simulink library "CTRL_LO"  (R2023b)
settings: Solver=VariableStepAuto  StartTime=0.0  StopTime=10.0  RelTol=1e-3
undefined symbols (not defined in the file or in its folder): CTRL_LO_p_SwtTqMotReqStrat_na
libraries: CTRL_LO_FRDIST x1, CTRL_LO_ST1 x1, CTRL_LO_ST2 x1, CTRL_LO_ST3 x1, CTRL_LO_ST4 x1, CTRL_LO_ST5 x1
settings Model: Creator=blatak  LastModifiedBy=blatak

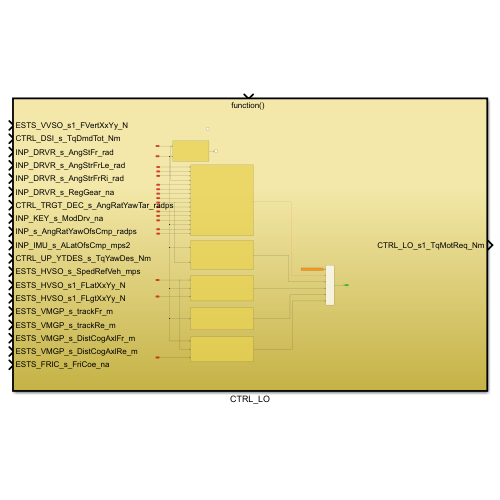
[thumbnail: Simulink's stored preview of the top-level diagram]
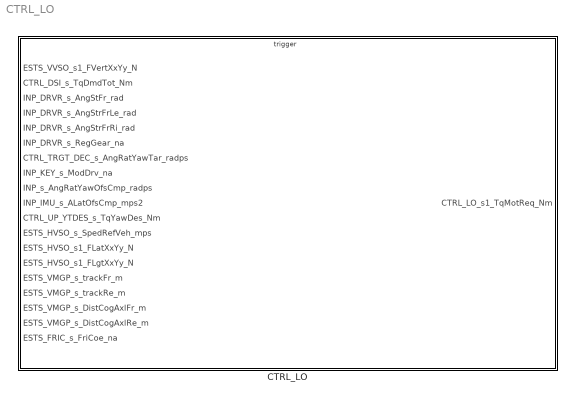
== system CTRL_LO ==
  CTRL_LO : Subsystem  TreatAsAtomicUnit=on

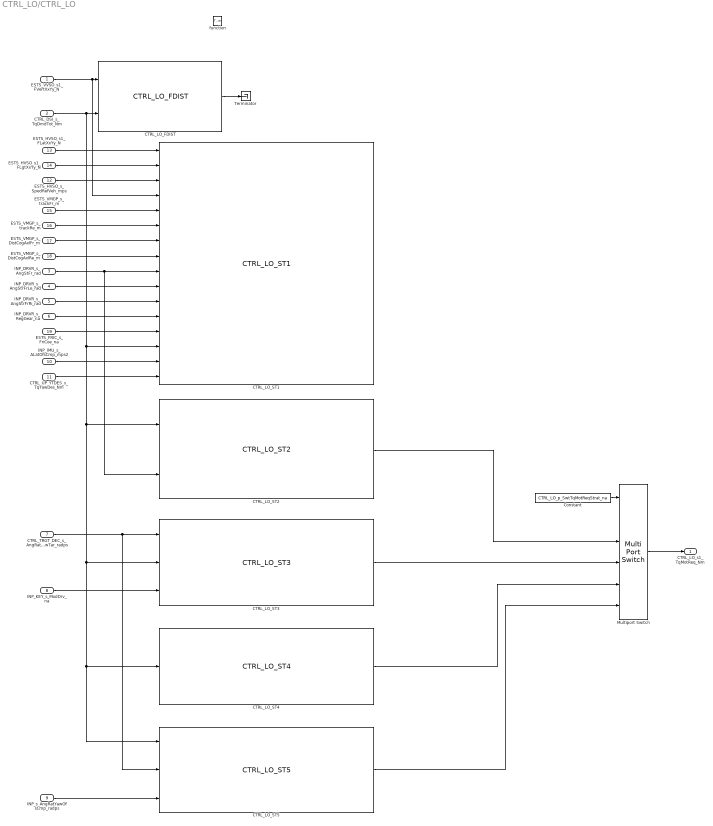
== system CTRL_LO/CTRL_LO ==
  ESTS_VVSO_s1_FVertXxYy_N : Inport
  CTRL_DSI_s_TqDmdTot_Nm : Inport  Port=2
  INP_DRVR_s_AngStFr_rad : Inport  Port=3
  INP_DRVR_s_AngStrFrLe_rad : Inport  Port=4
  INP_DRVR_s_AngStrFrRi_rad : Inport  Port=5
  INP_DRVR_s_RegGear_na : Inport  Port=6
  CTRL_TRGT_DEC_s_AngRatYawTar_radps : Inport  Port=7
  INP_KEY_s_ModDrv_na : Inport  Port=8
  INP_s_AngRatYawOfsCmp_radps : Inport  Port=9
  INP_IMU_s_ALatOfsCmp_mps2 : Inport  Port=10
  CTRL_UP_YTDES_s_TqYawDes_Nm : Inport  Port=11
  ESTS_HVSO_s_SpedRefVeh_mps : Inport  Port=12
  ESTS_HVSO_s1_FLatXxYy_N : Inport  Port=13
  ESTS_HVSO_s1_FLgtXxYy_N : Inport  Port=14
  ESTS_VMGP_s_trackFr_m : Inport  Port=15
  ESTS_VMGP_s_trackRe_m : Inport  Port=16
  ESTS_VMGP_s_DistCogAxlFr_m : Inport  Port=17
  ESTS_VMGP_s_DistCogAxlRe_m : Inport  Port=18
  ESTS_FRIC_s_FriCoe_na : Inport  Port=19
  function : TriggerPort  TriggerType=function-call  VariantControl=(inherit)
  CTRL_LO_FDIST : CTRL_LO_FRDIST/CTRL_LO_FDIST  SystemSampleTime=-1  VariantActivationTime=update diagram  AllowFlexibleInterface=on  Latency=0  AutoFrameSizeCalculation=off
  CTRL_LO_ST1 : CTRL_LO_ST1/CTRL_LO_ST1  SystemSampleTime=-1  VariantActivationTime=update diagram  AllowFlexibleInterface=on  Latency=0  AutoFrameSizeCalculation=off
  CTRL_LO_ST2 : CTRL_LO_ST2/CTRL_LO_ST2  SystemSampleTime=-1  VariantActivationTime=update diagram  AllowFlexibleInterface=on  Latency=0  AutoFrameSizeCalculation=off
  CTRL_LO_ST3 : CTRL_LO_ST3/CTRL_LO_ST3  SystemSampleTime=-1  VariantActivationTime=update diagram  AllowFlexibleInterface=on  Latency=0  AutoFrameSizeCalculation=off
  CTRL_LO_ST4 : CTRL_LO_ST4/CTRL_LO_ST4  SystemSampleTime=-1  VariantActivationTime=update diagram  AllowFlexibleInterface=on  Latency=0  AutoFrameSizeCalculation=off
  CTRL_LO_ST5 : CTRL_LO_ST5/CTRL_LO_ST5  SystemSampleTime=-1  VariantActivationTime=update diagram  AllowFlexibleInterface=on  Latency=0  AutoFrameSizeCalculation=off
  Constant : Constant  Value=CTRL_LO_p_SwtTqMotReqStrat_na
  Multiport Switch : MultiPortSwitch  Inputs=5  SaturateOnIntegerOverflow=off  InputSameDT=off
  Terminator : Terminator
  CTRL_LO_s1_TqMotReq_Nm : Outport
  wires:
  ESTS_VVSO_s1_FVertXxYy_N/1 -> CTRL_LO_ST1/4, CTRL_LO_FDIST/1
  CTRL_DSI_s_TqDmdTot_Nm/1 -> CTRL_LO_ST5/1, CTRL_LO_ST4/1, CTRL_LO_ST3/2, CTRL_LO_ST2/1, CTRL_LO_ST1/14, CTRL_LO_FDIST/2
  CTRL_LO_FDIST/1 -> Terminator/1
  ? -> Multiport Switch/2
  CTRL_LO_ST2/1 -> Multiport Switch/3
  CTRL_LO_ST3/1 -> Multiport Switch/4
  CTRL_LO_ST4/1 -> Multiport Switch/5
  CTRL_LO_ST5/1 -> Multiport Switch/6
  Multiport Switch/1 -> CTRL_LO_s1_TqMotReq_Nm/1
  INP_DRVR_s_AngStFr_rad/1 -> CTRL_LO_ST2/2, CTRL_LO_ST1/9
  CTRL_TRGT_DEC_s_AngRatYawTar_radps/1 -> CTRL_LO_ST5/2, CTRL_LO_ST3/1
  INP_KEY_s_ModDrv_na/1 -> CTRL_LO_ST3/3
  INP_s_AngRatYawOfsCmp_radps/1 -> CTRL_LO_ST5/3
  Constant/1 -> Multiport Switch/1
  CTRL_UP_YTDES_s_TqYawDes_Nm/1 -> CTRL_LO_ST1/16
  ESTS_HVSO_s1_FLatXxYy_N/1 -> CTRL_LO_ST1/1
  ESTS_HVSO_s1_FLgtXxYy_N/1 -> CTRL_LO_ST1/2
  ESTS_HVSO_s_SpedRefVeh_mps/1 -> CTRL_LO_ST1/3
  ESTS_VMGP_s_trackFr_m/1 -> CTRL_LO_ST1/5
  ESTS_VMGP_s_trackRe_m/1 -> CTRL_LO_ST1/6
  ESTS_VMGP_s_DistCogAxlFr_m/1 -> CTRL_LO_ST1/7
  ESTS_VMGP_s_DistCogAxlRe_m/1 -> CTRL_LO_ST1/8
  INP_DRVR_s_AngStrFrLe_rad/1 -> CTRL_LO_ST1/10
  INP_DRVR_s_AngStrFrRi_rad/1 -> CTRL_LO_ST1/11
  INP_DRVR_s_RegGear_na/1 -> CTRL_LO_ST1/12
  ESTS_FRIC_s_FriCoe_na/1 -> CTRL_LO_ST1/13
  INP_IMU_s_ALatOfsCmp_mps2/1 -> CTRL_LO_ST1/15
